simulink model "Ans8_Robo2_closedloop_feedback"  (R2022b)
settings: Solver=VariableStepAuto  StartTime=0.0  StopTime=10.0  RelTol=1e-3
undefined symbols (not defined in the file or in its folder): sigbuilder_block
settings Model: Creator=SysIDEA_OSACE  LastModifiedBy=SysIDEA_OSACE

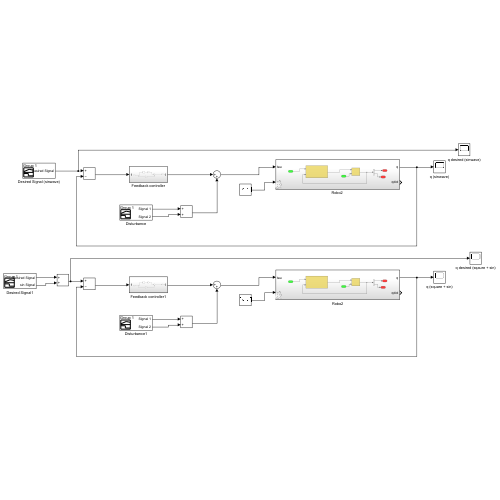
[thumbnail: Simulink's stored preview of the top-level diagram]
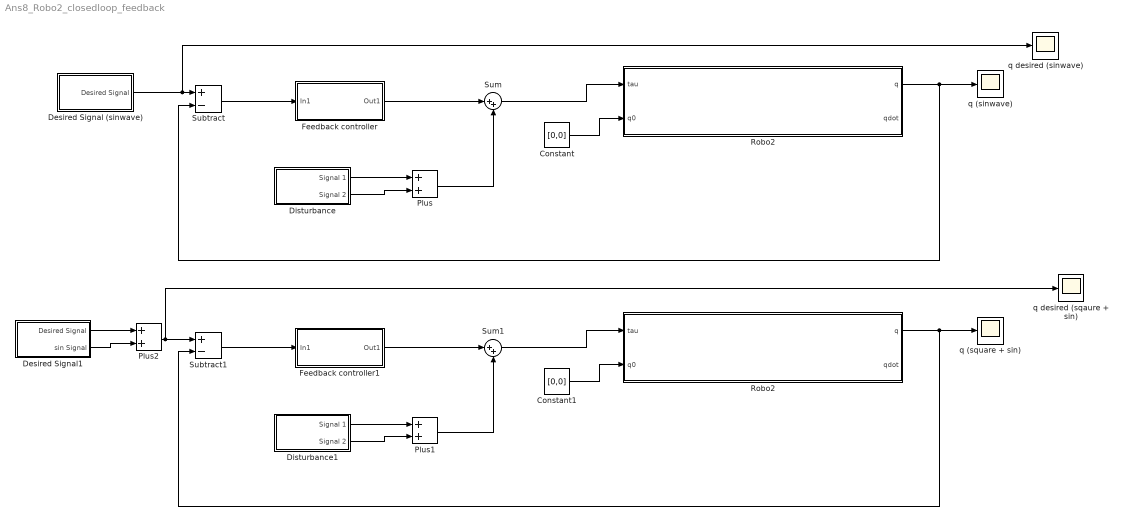
== system Ans8_Robo2_closedloop_feedback ==
  Constant : Constant  Value=[0,0]
  Constant1 : Constant  Value=[0,0]
  Desired Signal (sinwave) : Subsystem  Tag=STV Subsys  LoadFcn=sigbuilder_block('load');  StartFcn=sigbuilder_block('start');  StopFcn=sigbuilder_block('stop');  ClipboardFcn=sigbuilder_block('clipboard');  mask(Sigbuilder block){tuvar=[0:10]}
      mask help: Simulink:masks:SigbuilderBlock_MD
      mask init:
      | if ~strcmp(get_param(bdroot(gcbh),'SimulationStatus'),'stopped') tuvar = sigbuilder_block('maskInit'); end
      settings: CopyFcn=sigbuilder_block('copy');  DeleteFcn=sigbuilder_block('delete');  ModelCloseFcn=sigbuilder_block('modelClose');  PreSaveFcn=sigbuilder_block('preSave');  PauseFcn=sigbuilder_block('pause');  ContinueFcn=sigbuilder_block('continue');  NameChangeFcn=sigbuilder_block('namechange');  OpenFcn=sigbuilder_block('open',[437.6 199.2 550.4 400 ]);  CloseFcn=sigbuilder_block('close');
      mask Display: plot(0, 0, 100, 100,[2, 2, 32, 32, 2], [68, 8, 8, 68, 68],[32, 2], [38, 38], [32, 19, 2],[53, 60, 44], [32, 17, 17, 2],[16, 16, 31, 31]);txt = getActiveGroup(gcbh);text(2, 100, txt,'verticalAlignment', 'top');
  Desired Signal1 : Subsystem  Tag=STV Subsys  LoadFcn=sigbuilder_block('load');  StartFcn=sigbuilder_block('start');  StopFcn=sigbuilder_block('stop');  ClipboardFcn=sigbuilder_block('clipboard');  mask(Sigbuilder block){tuvar=[0:10]}
      mask help: Simulink:masks:SigbuilderBlock_MD
      mask init:
      | if ~strcmp(get_param(bdroot(gcbh),'SimulationStatus'),'stopped') tuvar = sigbuilder_block('maskInit'); end
      settings: CopyFcn=sigbuilder_block('copy');  DeleteFcn=sigbuilder_block('delete');  ModelCloseFcn=sigbuilder_block('modelClose');  PreSaveFcn=sigbuilder_block('preSave');  PauseFcn=sigbuilder_block('pause');  ContinueFcn=sigbuilder_block('continue');  NameChangeFcn=sigbuilder_block('namechange');  OpenFcn=sigbuilder_block('open',[437.6 199.2 550.4 400 ]);  CloseFcn=sigbuilder_block('close');
      mask Display: plot(0, 0, 100, 100,[2, 2, 32, 32, 2], [68, 8, 8, 68, 68],[32, 2], [38, 38], [32, 19, 2],[53, 60, 44], [32, 17, 17, 2],[16, 16, 31, 31]);txt = getActiveGroup(gcbh);text(2, 100, txt,'verticalAlignment', 'top');
  Disturbance : Subsystem  Tag=STV Subsys  LoadFcn=sigbuilder_block('load');  StartFcn=sigbuilder_block('start');  StopFcn=sigbuilder_block('stop');  ClipboardFcn=sigbuilder_block('clipboard');  mask(Sigbuilder block){tuvar=[0:10]}
      mask help: Simulink:masks:SigbuilderBlock_MD
      mask init:
      | if ~strcmp(get_param(bdroot(gcbh),'SimulationStatus'),'stopped') tuvar = sigbuilder_block('maskInit'); end
      settings: CopyFcn=sigbuilder_block('copy');  DeleteFcn=sigbuilder_block('delete');  ModelCloseFcn=sigbuilder_block('modelClose');  PreSaveFcn=sigbuilder_block('preSave');  PauseFcn=sigbuilder_block('pause');  ContinueFcn=sigbuilder_block('continue');  NameChangeFcn=sigbuilder_block('namechange');  OpenFcn=sigbuilder_block('open',[437.6 199.2 550.4 400 ]);  CloseFcn=sigbuilder_block('close');
      mask Display: plot(0, 0, 100, 100,[2, 2, 32, 32, 2], [68, 8, 8, 68, 68],[32, 2], [38, 38], [32, 19, 2],[53, 60, 44], [32, 17, 17, 2],[16, 16, 31, 31]);txt = getActiveGroup(gcbh);text(2, 100, txt,'verticalAlignment', 'top');
  Disturbance1 : Subsystem  Tag=STV Subsys  LoadFcn=sigbuilder_block('load');  StartFcn=sigbuilder_block('start');  StopFcn=sigbuilder_block('stop');  ClipboardFcn=sigbuilder_block('clipboard');  mask(Sigbuilder block){tuvar=[0:10]}
      mask help: Simulink:masks:SigbuilderBlock_MD
      mask init:
      | if ~strcmp(get_param(bdroot(gcbh),'SimulationStatus'),'stopped') tuvar = sigbuilder_block('maskInit'); end
      settings: CopyFcn=sigbuilder_block('copy');  DeleteFcn=sigbuilder_block('delete');  ModelCloseFcn=sigbuilder_block('modelClose');  PreSaveFcn=sigbuilder_block('preSave');  PauseFcn=sigbuilder_block('pause');  ContinueFcn=sigbuilder_block('continue');  NameChangeFcn=sigbuilder_block('namechange');  OpenFcn=sigbuilder_block('open',[437.6 199.2 550.4 400 ]);  CloseFcn=sigbuilder_block('close');
      mask Display: plot(0, 0, 100, 100,[2, 2, 32, 32, 2], [68, 8, 8, 68, 68],[32, 2], [38, 38], [32, 19, 2],[53, 60, 44], [32, 17, 17, 2],[16, 16, 31, 31]);txt = getActiveGroup(gcbh);text(2, 100, txt,'verticalAlignment', 'top');
  Feedback controller : Subsystem
  Feedback controller1 : Subsystem
  Plus : Sum
  Plus1 : Sum
  Plus2 : Sum
  Robo2 : Subsystem  AncestorBlock=mssSimulink/Marine craft models/Remus 100 AUV (remus100.m)
      settings: LibrarySourceBlock=mssSimulink/Marine craft models/Remus 100 AUV (remus100.m)
  "Robo2 " : Subsystem  AncestorBlock=mssSimulink/Marine craft models/Remus 100 AUV (remus100.m)
      settings: LibrarySourceBlock=mssSimulink/Marine craft models/Remus 100 AUV (remus100.m)
  Subtract : Sum  Inputs=+-
  Subtract1 : Sum  Inputs=+-
  Sum : Sum  Inputs=|++
  Sum1 : Sum  Inputs=|++
  q (sinwave) : Scope
  q (square + sin) : Scope
  q desired (sinwave) : Scope
  q desired (sqaure + sin) : Scope
  wires:
  Robo2/1(q) -> Subtract1/2, q (square + sin)/1
  Desired Signal1/2(sin Signal) -> Plus2/2
  Desired Signal (sinwave)/1(Desired Signal) -> q desired (sinwave)/1, Subtract/1
  Desired Signal1/1(Desired Signal) -> Plus2/1
  Constant1/1 -> Robo2/2(q0)
  Plus1/1 -> Sum1/2
  Feedback controller1/1(Out1) -> Sum1/1
  Subtract1/1 -> Feedback controller1/1(In1)
  Disturbance1/1(Signal 1) -> Plus1/1
  Disturbance/2(Signal 2) -> Plus/2
  Sum1/1 -> Robo2/1(tau)
  Constant/1 -> "Robo2 "/2(q0)
  Disturbance1/2(Signal 2) -> Plus1/2
  Sum/1 -> "Robo2 "/1(tau)
  Plus/1 -> Sum/2
  Subtract/1 -> Feedback controller/1(In1)
  Disturbance/1(Signal 1) -> Plus/1
  Feedback controller/1(Out1) -> Sum/1
  Plus2/1 -> q desired (sqaure + sin)/1, Subtract1/1
  "Robo2 "/1(q) -> Subtract/2, q (sinwave)/1

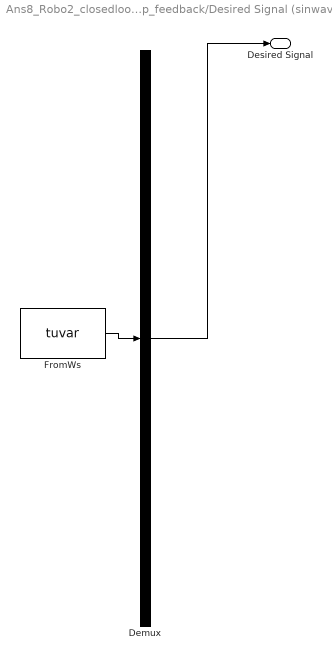
== system Ans8_Robo2_closedloop_feedback/Desired Signal (sinwave) ==
  Demux : Demux  Tag=STV Demux  Outputs=1
      settings: DisplayOption=none
  FromWs : FromWorkspace  Tag=STV FromWs  VariableName=tuvar
      SigBuilderData=|
      | common.afterFinalStr = 'Extrapolate'
      | common.sampleTime = 0
      | dataSet.timeRange = [0 10]
      | dataSet.name = 'Group 1'
      | sbobj.Groups.Name = 'Group 1'
      | sbobj.Groups.Signals.Name = 'Desired Signal'
      | sbobj.Groups.Signals.XData = [0 0.125 0.25 0.375 0.5 0.625 0.75 0.875 1 1.125 1.25 1.375 1.5 1.625 1.75 1.875 2 2.125 2.25 2.375 2.5 2.625 2.75 2.875 3 3.125 3.25 3.375 3.5 3.625 3.75 3.875 4 4.125 4.25 4.375 4.5 4.625 4.75 4.875 5 5.125 5.25 5.375 5.5 5.625 5.75 5.875 6 6.125 6.25 6.375 6.5 6.625 6.75 6.875 7 7.125 7.25 7.375 7.5 7.625 7.75 7.875 8 8.125 8.25 8.375 8.5 8.625 8.75 8.875 9 9.125 9.25 9.375 9.5 9.625 9.75 9.875 10]
      | sbobj.Groups.Signals.YData = [1 71.7106781187 101 71.7106781187 1 -69.7106781187 -99 -69.7106781187 1 71.7106781187 101 71.7106781187 1 -69.7106781187 -99 -69.7106781187 1 71.7106781187 101 71.7106781187 1 -69.7106781187 -99 -69.7106781187 1 71.7106781187 101 71.7106781187 1 -69.7106781187 -99 -69.7106781187 1 71.7106781187 101 71.7106781187 1 -69.7106781187 -99 -69.7106781187 1 71.7106781187 101 71.7106781187 1 -69.7106781187 -99 -69.7106781187 1 71.7106781187 101 71.7106781187 1 -69.7106781187 -99 -69.7106781187 1 71.7106781187 101 71.7106781187 1 -69.7106781187 -99 -69.7106781187 1 71.7106781187 101 71.7106781187 1 -69.7106781187 -99 -69.7106781187 1 71.7106781187 101 71.7106781187 1 -69.7106781187 -99 -69.7106781187 1]
  Desired Signal : Outport  Tag=STV Outport
  wires:
  FromWs/1 -> Demux/1
  Demux/1 -> Desired Signal/1

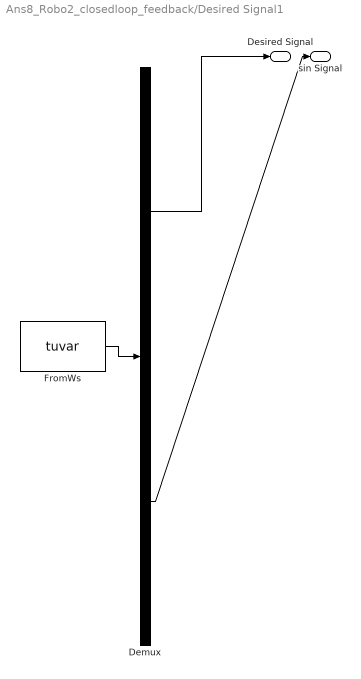
== system Ans8_Robo2_closedloop_feedback/Desired Signal1 ==
  Demux : Demux  Tag=STV Demux  Outputs=2
      settings: DisplayOption=none
  FromWs : FromWorkspace  Tag=STV FromWs  VariableName=tuvar
      SigBuilderData=|
      | common.afterFinalStr = 'Extrapolate'
      | common.sampleTime = 0
      | dataSet.timeRange = [0 10]
      | dataSet.name = 'Group 1'
      | sbobj.Groups.Name = 'Group 1'
      | sbobj.Groups.Signals(1).Name = 'Desired Signal'
      | sbobj.Groups.Signals(1).XData = [0 0.5 0.5 1 1 1.5 1.5 2 2 2.5 2.5 3 3 3.5 3.5 4 4 4.5 4.5 5 5 5.5 5.5 6 6 6.5 6.5 7 7 7.5 7.5 8 8 8.5 8.5 9 9 9.5 9.5 10]
      | sbobj.Groups.Signals(1).YData = [100 100 0 0 100 100 0 0 100 100 0 0 100 100 0 0 100 100 0 0 100 100 0 0 100 100 0 0 100 100 0 0 100 100 0 0 100 100 0 0]
      | sbobj.Groups.Signals(2).Name = 'sin Signal'
      | sbobj.Groups.Signals(2).XData = [0 0.125 0.25 0.375 0.5 0.625 0.75 0.875 1 1.125 1.25 1.375 1.5 1.625 1.75 1.875 2 2.125 2.25 2.375 2.5 2.625 2.75 2.875 3 3.125 3.25 3.375 3.5 3.625 3.75 3.875 4 4.125 4.25 4.375 4.5 4.625 4.75 4.875 5 5.125 5.25 5.375 5.5 5.625 5.75 5.875 6 6.125 6.25 6.375 6.5 6.625 6.75 6.875 7 7.125 7.25 7.375 7.5 7.625 7.75 7.875 8 8.125 8.25 8.375 8.5 8.625 8.75 8.875 9 9.125 9.25 9.375 9.5 9.625 9.75 9.875 10]
      | sbobj.Groups.Signals(2).YData = [50 64.1421356237 70 64.1421356237 50 35.8578643763 30 35.8578643763 50 64.1421356237 70 64.1421356237 50 35.8578643763 30 35.8578643763 50 64.1421356237 70 64.1421356237 50 35.8578643763 30 35.8578643763 50 64.1421356237 70 64.1421356237 50 35.8578643763 30 35.8578643763 50 64.1421356237 70 64.1421356237 50 35.8578643763 30 35.8578643763 50 64.1421356237 70 64.1421356237 50 35.8578643763 30 35.8578643763 50 64.1421356237 70 64.1421356237 50 35.8578643763 30 35.8578643763 50 64.1421356237 70 64.1421356237 50 35.8578643763 30 35.8578643763 50 64.1421356237 70 64.1421356237 50 35.8578643763 30 35.8578643763 50 64.1421356237 70 64.1421356237 50 35.8578643763 30 35.8578643763 50]
  Desired Signal : Outport  Tag=STV Outport
  sin Signal : Outport  Tag=STV Outport  Port=2
  wires:
  FromWs/1 -> Demux/1
  Demux/1 -> Desired Signal/1
  Demux/2 -> sin Signal/1

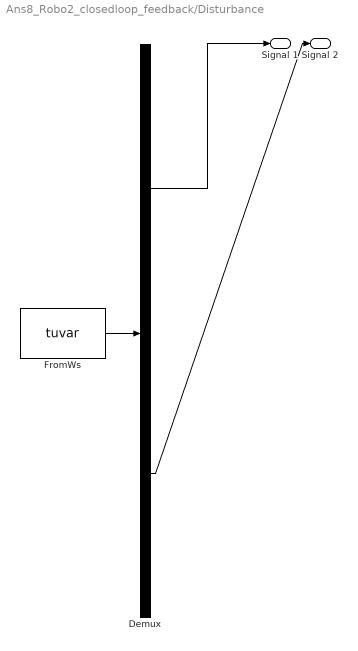
== system Ans8_Robo2_closedloop_feedback/Disturbance ==
  Demux : Demux  Tag=STV Demux  Outputs=2
      settings: DisplayOption=none
  FromWs : FromWorkspace  Tag=STV FromWs  VariableName=tuvar
      SigBuilderData=|
      | common.afterFinalStr = 'Extrapolate'
      | common.sampleTime = 0
      | dataSet.timeRange = [0 10]
      | dataSet.name = 'Group 1'
      | sbobj.Groups.Name = 'Group 1'
      | sbobj.Groups.Signals(1).Name = 'Signal 1'
      | sbobj.Groups.Signals(1).XData = [0 1.42 1.42 6 6 10]
      | sbobj.Groups.Signals(1).YData = [0 0 23 23 0 0]
      | sbobj.Groups.Signals(2).Name = 'Signal 2'
      | sbobj.Groups.Signals(2).XData = [0 0.1 0.2 0.3 0.4 0.5 0.6 0.7 0.8 0.9 1 1.1 1.2 1.3 1.4 1.5 1.6 1.7 1.8 1.9 2 2.1 2.2 2.3 2.4 2.5 2.6 2.7 2.8 2.9 3 3.1 3.2 3.3 3.4 3.5 3.6 3.7 3.8 3.9 4 4.1 4.2 4.3 4.4 4.5 4.6 4.7 4.8 4.9 5 5.1 5.2 5.3 5.4 5.5 5.6 5.7 5.8 5.9 6 6.1 6.2 6.3 6.4 6.5 6.6 6.7 6.8 6.9 7 7.1 7.2 7.3 7.4 7.5 7.6 7.7 7.8 7.9 8 8.1 8.2 8.3 8.4 8.5 8.6 8.7 8.8 8.9 9 9.1 9.2 9.3 9.4 9.5 9.6 9.7 9.8 9.9 10]
      | sbobj.Groups.Signals(2).YData = [1.0570332669 -0.216920199324 -0.152501941548 0.700051897858 0.565756771412 -1.11025500149 -1.52269301393 -1.08786776954 -1.40577332157 0.069570588566 -0.401250925532 -0.358010733041 -1.35096312939 0.789567428735 0.449411111554 -0.0796224837412 1.03118011801 -0.863979465029 0.424700293048 0.358441199952 0.359254416664 -0.71924726763 0.336840248763 -0.504881632926 -0.886446150502 -1.19326818642 1.04781563949 -0.835944212336 -0.162913844259 -1.19865205474 -0.287126799995 -3.22203779594 -1.07695922946 -1.41643615948 -1.00445076771 -0.203267188307 -0.31534778036 6.5 -0.561773218349 -0.240032278035 -1.55931547034 -0.467382663694 -1.32797665356 0.0402990237882 0.863086767519 0.414253465109 -0.690620213418 -1.62054289275 1.47001318514 2.06004273294 0.130500599699 -0.979901604221 1.20777147431 -0.582656218169 -0.459809363224 0.896377377073 -1.37521980111 -1.94675395423 0.430683700201 0.410737998147 0.105142157864 0.506684391637 1.09224059616 0.980447788355 -0.55856957039 0.819972073319 0.183247371832 -0.495542568515 -1.18330579089 0.656970938881 -0.343622599299 0.0564345266878 -0.782947502202 -1.54051447478 0.181586355269 -0.0521391248044 1.20902787729 0.811704070327 1.06330457915 -0.738876752543 -0.926326497116 -1.25908677287 0.507980623047 2.79908112764 0.737572036916 -0.763064102152 0.846633754476 -1.11833031008 -1.41447009142 0.727442315507 -0.767905520185 0.325985880709 1.41653513808 0.411124635732 0.93966028442 -1.59580220462 0.671536244123 2.14850225383 0.551139413417 -1.53087718186 -0.193142794822]
  Signal 1 : Outport  Tag=STV Outport
  Signal 2 : Outport  Tag=STV Outport  Port=2
  wires:
  Demux/1 -> Signal 1/1
  FromWs/1 -> Demux/1
  Demux/2 -> Signal 2/1

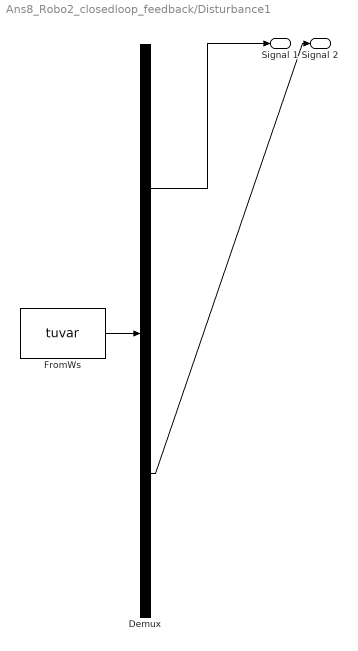
== system Ans8_Robo2_closedloop_feedback/Disturbance1 ==
  Demux : Demux  Tag=STV Demux  Outputs=2
      settings: DisplayOption=none
  FromWs : FromWorkspace  Tag=STV FromWs  VariableName=tuvar
      SigBuilderData=|
      | common.afterFinalStr = 'Extrapolate'
      | common.sampleTime = 0
      | dataSet.timeRange = [0 10]
      | dataSet.name = 'Group 1'
      | sbobj.Groups.Name = 'Group 1'
      | sbobj.Groups.Signals(1).Name = 'Signal 1'
      | sbobj.Groups.Signals(1).XData = [0 1.42 1.42 6 6 10]
      | sbobj.Groups.Signals(1).YData = [0 0 23 23 0 0]
      | sbobj.Groups.Signals(2).Name = 'Signal 2'
      | sbobj.Groups.Signals(2).XData = [0 0.1 0.2 0.3 0.4 0.5 0.6 0.7 0.8 0.9 1 1.1 1.2 1.3 1.4 1.5 1.6 1.7 1.8 1.9 2 2.1 2.2 2.3 2.4 2.5 2.6 2.7 2.8 2.9 3 3.1 3.2 3.3 3.4 3.5 3.6 3.7 3.8 3.9 4 4.1 4.2 4.3 4.4 4.5 4.6 4.7 4.8 4.9 5 5.1 5.2 5.3 5.4 5.5 5.6 5.7 5.8 5.9 6 6.1 6.2 6.3 6.4 6.5 6.6 6.7 6.8 6.9 7 7.1 7.2 7.3 7.4 7.5 7.6 7.7 7.8 7.9 8 8.1 8.2 8.3 8.4 8.5 8.6 8.7 8.8 8.9 9 9.1 9.2 9.3 9.4 9.5 9.6 9.7 9.8 9.9 10]
      | sbobj.Groups.Signals(2).YData = [1.0570332669 -0.216920199324 -0.152501941548 0.700051897858 0.565756771412 -1.11025500149 -1.52269301393 -1.08786776954 -1.40577332157 0.069570588566 -0.401250925532 -0.358010733041 -1.35096312939 0.789567428735 0.449411111554 -0.0796224837412 1.03118011801 -0.863979465029 0.424700293048 0.358441199952 0.359254416664 -0.71924726763 0.336840248763 -0.504881632926 -0.886446150502 -1.19326818642 1.04781563949 -0.835944212336 -0.162913844259 -1.19865205474 -0.287126799995 -3.22203779594 -1.07695922946 -1.41643615948 -1.00445076771 -0.203267188307 -0.31534778036 6.5 -0.561773218349 -0.240032278035 -1.55931547034 -0.467382663694 -1.32797665356 0.0402990237882 0.863086767519 0.414253465109 -0.690620213418 -1.62054289275 1.47001318514 2.06004273294 0.130500599699 -0.979901604221 1.20777147431 -0.582656218169 -0.459809363224 0.896377377073 -1.37521980111 -1.94675395423 0.430683700201 0.410737998147 0.105142157864 0.506684391637 1.09224059616 0.980447788355 -0.55856957039 0.819972073319 0.183247371832 -0.495542568515 -1.18330579089 0.656970938881 -0.343622599299 0.0564345266878 -0.782947502202 -1.54051447478 0.181586355269 -0.0521391248044 1.20902787729 0.811704070327 1.06330457915 -0.738876752543 -0.926326497116 -1.25908677287 0.507980623047 2.79908112764 0.737572036916 -0.763064102152 0.846633754476 -1.11833031008 -1.41447009142 0.727442315507 -0.767905520185 0.325985880709 1.41653513808 0.411124635732 0.93966028442 -1.59580220462 0.671536244123 2.14850225383 0.551139413417 -1.53087718186 -0.193142794822]
  Signal 1 : Outport  Tag=STV Outport
  Signal 2 : Outport  Tag=STV Outport  Port=2
  wires:
  Demux/1 -> Signal 1/1
  FromWs/1 -> Demux/1
  Demux/2 -> Signal 2/1

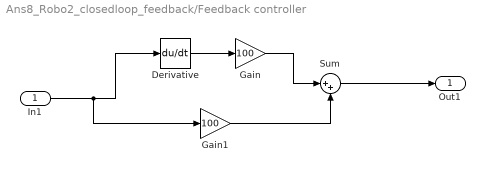
== system Ans8_Robo2_closedloop_feedback/Feedback controller ==
  In1 : Inport
  Derivative : Derivative
  Gain : Gain  Gain=100
  Gain1 : Gain  Gain=100
  Sum : Sum  Inputs=|++
  Out1 : Outport
  wires:
  In1/1 -> Derivative/1, Gain1/1
  Sum/1 -> Out1/1
  Derivative/1 -> Gain/1
  Gain/1 -> Sum/1
  Gain1/1 -> Sum/2

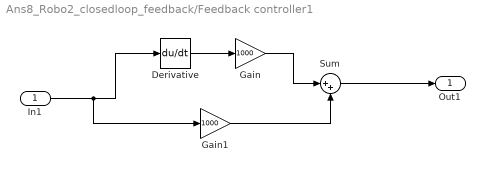
== system Ans8_Robo2_closedloop_feedback/Feedback controller1 ==
  In1 : Inport
  Derivative : Derivative
  Gain : Gain  Gain=1000
  Gain1 : Gain  Gain=1000
  Sum : Sum  Inputs=|++
  Out1 : Outport
  wires:
  In1/1 -> Derivative/1, Gain1/1
  Sum/1 -> Out1/1
  Derivative/1 -> Gain/1
  Gain/1 -> Sum/1
  Gain1/1 -> Sum/2

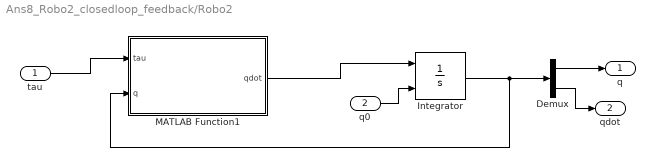
== system Ans8_Robo2_closedloop_feedback/Robo2 ==
  tau : Inport
  q0 : Inport  Port=2
  Demux : Demux  Outputs=2
  Integrator : Integrator  InitialConditionSource=external  InitialCondition=[1 1]  UpperSaturationLimit=10  LowerSaturationLimit=-10
  MATLAB Function1 : MATLAB Function  TreatAsAtomicUnit=on
  q : Outport
  qdot : Outport  Port=2
  wires:
  MATLAB Function1/1(qdot) -> Integrator/1
  q0/1 -> Integrator/2
  Integrator/1 -> Demux/1, MATLAB Function1/2(q)
  tau/1 -> MATLAB Function1/1(tau)
  Demux/1 -> q/1
  Demux/2 -> qdot/1

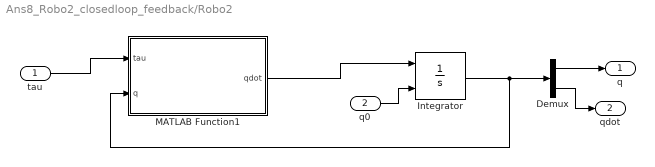
== system Ans8_Robo2_closedloop_feedback/Robo2  ==
  tau : Inport
  q0 : Inport  Port=2
  Demux : Demux  Outputs=2
  Integrator : Integrator  InitialConditionSource=external  InitialCondition=[1 1]  UpperSaturationLimit=10  LowerSaturationLimit=-10
  MATLAB Function1 : MATLAB Function  TreatAsAtomicUnit=on
  q : Outport
  qdot : Outport  Port=2
  wires:
  MATLAB Function1/1(qdot) -> Integrator/1
  q0/1 -> Integrator/2
  Integrator/1 -> Demux/1, MATLAB Function1/2(q)
  tau/1 -> MATLAB Function1/1(tau)
  Demux/1 -> q/1
  Demux/2 -> qdot/1

== matlab function Ans8_Robo2_closedloop_feedback/Robo2 /MATLAB Function1 ==
  data: tau input; qdot output; q input
function qdot  = fcn(tau,q)

  [qdot] = Robo2(tau,q);

end

== matlab function Ans8_Robo2_closedloop_feedback/Robo2/MATLAB Function1 ==
  data: tau input; qdot output; q input
function qdot  = fcn(tau,q)

  [qdot] = Robo2(tau,q);

end
